simulink model "simple"  (R2019b)
settings: Solver=VariableStepAuto  StartTime=0.0  StopTime=10.0  RelTol=1e-3
values from neighbouring files (symbols this model uses):
  g = 9.81    [G.m]    (also in connect_pend_runner.m = -9.81; run.m; single_pend_runner.m = -9.81)
  Kd = 50    [anujay_single_pendulum_same.m]    (also in connect_pend_runner.m = 10; double_pend_setup.m = [50,0;0,50]; run.m = 300; single_pend_runner.m = 500)
  Kd_imped = 10000    [run.m]
  Kp = 300    [run.m]    (also in single_pend_runner.m = 500)
  Kp_imped = 10000    [run.m]
  l = [ 1.0, 1.5]    [double_pend_setup.m]    (also in run.m = 2)
  m = 10    [run.m]
libraries: robotcorelib x1
settings Model: Creator=nathanielgoldfarb  LastModifiedBy=nathanielgoldfarb

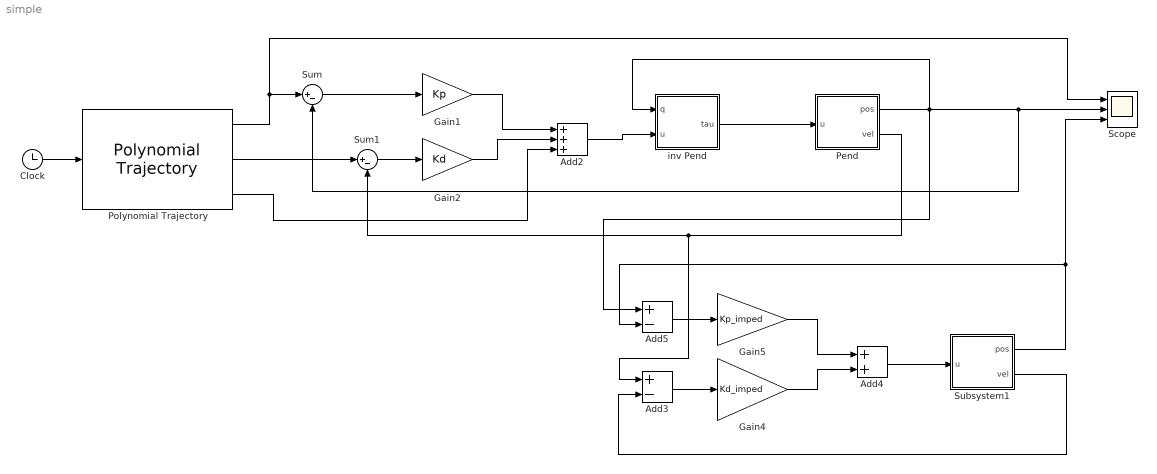
== system simple ==
  Add2 : Sum  Inputs=+++
  Add3 : Sum  Inputs=+-
  Add4 : Sum
  Add5 : Sum  Inputs=+-
  Clock : Clock
  Gain1 : Gain  Gain=Kp
  Gain2 : Gain  Gain=Kd
  Gain4 : Gain  Gain=Kd_imped
  Gain5 : Gain  Gain=Kp_imped
  Pend : Subsystem
  Polynomial Trajectory : robotcorelib/Polynomial Trajectory  WaypointSource=Internal  Waypoints=[ -pi , 0 ]  TimePoints=[ 0, 3]  TimeInterval=[ 1, 4 ]  Method=Cubic Polynomial  ParameterSource=Internal  VelocityBoundaryCondition=zeros( 1, 2 )  AccelerationBoundaryCondition=zeros( 2, 5 )  SimulateUsing=Interpreted execution
      settings: SourceProductName=Robotics System Toolbox  SourceProductBaseCode=RO
  Scope : Scope  NumInputPorts=3
  Subsystem1 : Subsystem
  Sum : Sum  Inputs=|+-
  Sum1 : Sum  Inputs=|+-
  inv Pend : Subsystem
  wires:
  Sum/1 -> Gain1/1
  Clock/1 -> Polynomial Trajectory/1
  Polynomial Trajectory/1 -> Scope/1, Sum/1
  Polynomial Trajectory/2 -> Sum1/1
  Sum1/1 -> Gain2/1
  Gain1/1 -> Add2/1
  Gain2/1 -> Add2/2
  Polynomial Trajectory/3 -> Add2/3
  Pend/1(pos) -> inv Pend/1(q), Scope/2, Sum/2, Add5/1
  Pend/2(vel) -> Add3/1, Sum1/2
  Add3/1 -> Gain4/1
  Gain4/1 -> Add4/2
  Add5/1 -> Gain5/1
  Gain5/1 -> Add4/1
  Add4/1 -> Subsystem1/1("u ")
  Subsystem1/1(pos) -> Scope/3, Add5/2
  Subsystem1/2(vel) -> Add3/2
  Add2/1 -> inv Pend/2("u ")
  inv Pend/1("tau ") -> Pend/1("u ")

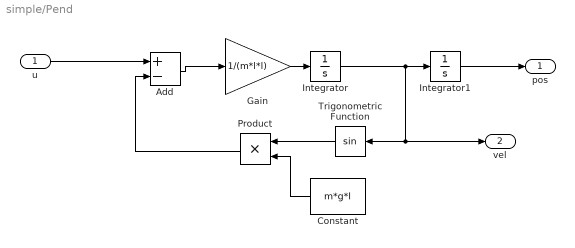
== system simple/Pend ==
  "u " : Inport
  Add : Sum  Inputs=+-
  Constant : Constant  Value=m*g*l
  Gain : Gain  Gain=1/(m*l*l)
  Integrator : Integrator
  Integrator1 : Integrator  InitialCondition=-pi
  Product : Product
  Trigonometric Function : Trigonometry
  pos : Outport
  vel : Outport  Port=2
  wires:
  Integrator1/1 -> pos/1
  "u "/1 -> Add/1
  Constant/1 -> Product/2
  Add/1 -> Gain/1
  Trigonometric Function/1 -> Product/1
  Product/1 -> Add/2
  Gain/1 -> Integrator/1
  Integrator/1 -> vel/1, Trigonometric Function/1, Integrator1/1

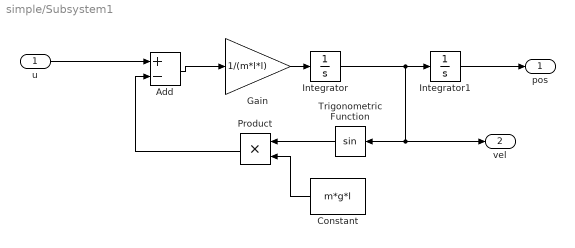
== system simple/Subsystem1 ==
  "u " : Inport
  Add : Sum  Inputs=+-
  Constant : Constant  Value=m*g*l
  Gain : Gain  Gain=1/(m*l*l)
  Integrator : Integrator
  Integrator1 : Integrator  InitialCondition=-pi
  Product : Product
  Trigonometric Function : Trigonometry
  pos : Outport
  vel : Outport  Port=2
  wires:
  Integrator1/1 -> pos/1
  "u "/1 -> Add/1
  Constant/1 -> Product/2
  Add/1 -> Gain/1
  Trigonometric Function/1 -> Product/1
  Product/1 -> Add/2
  Gain/1 -> Integrator/1
  Integrator/1 -> vel/1, Trigonometric Function/1, Integrator1/1

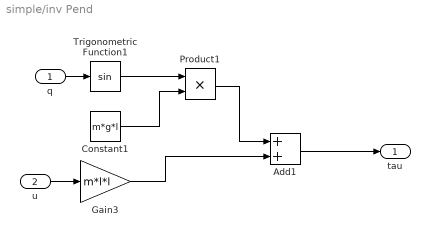
== system simple/inv Pend ==
  q : Inport
  "u " : Inport  Port=2
  Add1 : Sum
  Constant1 : Constant  Value=m*g*l
  Gain3 : Gain  Gain=m*l*l
  Product1 : Product
  Trigonometric Function1 : Trigonometry
  "tau " : Outport
  wires:
  Product1/1 -> Add1/1
  Constant1/1 -> Product1/2
  Add1/1 -> "tau "/1
  Gain3/1 -> Add1/2
  "u "/1 -> Gain3/1
  Trigonometric Function1/1 -> Product1/1
  q/1 -> Trigonometric Function1/1
